simulink model "final_quadruped_080722_support_polygon"  (R2021a)
settings: Solver=ode15s  StartTime=0.0  StopTime=10  FixedStep=1e-3  RelTol=1e-5  EnableMultiTasking=on
values from neighbouring files (symbols this model uses):
  foot_x = 8    [bipedparameters.m]    (also in fcn.m; finalrobotParameters.m; finalrobotParameters_110522.m; finalrobotParameters_140522.m)
  foot_y = 6    [bipedparameters.m]    (also in fcn.m; finalrobotParameters.m; finalrobotParameters_110522.m; finalrobotParameters_140522.m)
  foot_z = 1    [bipedparameters.m]    (also in fcn.m; finalrobotParameters.m; finalrobotParameters_110522.m; finalrobotParameters_140522.m)
  height_plane = 0.025    [bipedparameters.m]    (also in finalrobotParameters.m; finalrobotParameters_110522.m; finalrobotParameters_140522.m; finalrobotParameters_240522.m)
  kd_ankle = 1000    [bipedparameters.m]    (also in finalrobotParameters_240522.m)
  kd_hip = 1000    [bipedparameters.m]    (also in finalrobotParameters_240522.m)
  kd_knee = 1000    [bipedparameters.m]    (also in finalrobotParameters_240522.m)
  ki_ankle = 1000    [bipedparameters.m]    (also in finalrobotParameters_240522.m)
  ki_hip = 1000    [bipedparameters.m]    (also in finalrobotParameters_240522.m)
  ki_knee = 2000    [bipedparameters.m]    (also in finalrobotParameters_240522.m)
  kp_ankle = 1000    [bipedparameters.m]    (also in finalrobotParameters_240522.m)
  kp_hip = 1000    [bipedparameters.m]    (also in finalrobotParameters_240522.m)
  kp_knee = 2000    [bipedparameters.m]    (also in finalrobotParameters_240522.m)
  lower_leg_length = 10    [bipedparameters.m]    (also in fcn.m; finalrobotParameters.m; finalrobotParameters_110522.m; finalrobotParameters_140522.m)
  plane_x = 25    [bipedparameters.m]    (also in finalrobotParameters.m; finalrobotParameters_110522.m; finalrobotParameters_140522.m; finalrobotParameters_240522.m)
  plane_y = 3    [bipedparameters.m]    (also in finalrobotParameters.m; finalrobotParameters_110522.m; finalrobotParameters_140522.m; finalrobotParameters_240522.m)
  torso_offset_x = -0.5    [bipedparameters.m]    (also in finalrobotParameters.m = 10; finalrobotParameters_110522.m = 10; finalrobotParameters_140522.m = 10; finalrobotParameters_240522.m = 10)
  torso_offset_z = -2    [bipedparameters.m]    (also in finalrobotParameters.m; finalrobotParameters_110522.m; finalrobotParameters_140522.m; finalrobotParameters_240522.m)
  torso_x = 5    [bipedparameters.m]    (also in fcn.m = 25; finalrobotParameters.m = 25; finalrobotParameters_110522.m = 25; finalrobotParameters_140522.m = 25)
  torso_y = 10    [bipedparameters.m]    (also in fcn.m = 16; finalrobotParameters.m = 16; finalrobotParameters_110522.m = 16; finalrobotParameters_140522.m = 16)
  torso_z = 8    [bipedparameters.m]    (also in fcn.m = 10; finalrobotParameters.m = 10; finalrobotParameters_110522.m = 10; finalrobotParameters_140522.m = 10)
  upper_leg_length = 10    [bipedparameters.m]    (also in fcn.m; finalrobotParameters.m; finalrobotParameters_110522.m; finalrobotParameters_140522.m)
undefined symbols (not defined in the file or in its folder): sigbuilder_block, X, Y, Z
libraries: nesl_utility x288, sm_lib x71, pid_lib x20, Contact_Forces_Lib x16, fl_lib x3
(part 9 of 9)

== matlab function final_quadruped_080722_support_polygon/Model/Left Leg Back/Subsystem/MATLAB Function4 ==
  data: ed1g input; ed2g input; ed_dg1 output; ed_dg2 output; ed3g input; ed_dg3 output; ed4g input; ad3g input; ad4g input; ed5g input; vlinks input; w_torso input; ed_dg4 output; td123 input; v_torso input; ed_dg5 output; td4 input; td5 input; rho_dotLB output
function [ed_dg1,ed_dg2,ed_dg3,ed_dg4,ed_dg5,rho_dotLB] = fcn(ed1g,ed2g,ed3g,ed4g,ad3g,ad4g, ed5g, vlinks, w_torso, td123, v_torso, td4, td5)
w0=w_torso;
w1=w0*td123(1);
w2=w1*td123(2);
w3=w2+ed3g*td123(3);
w4=w3+ed4g*td4;
w5=w4+ed5g*td5;

%e dot = omega X e
ed_dg1=cross(w1,ed1g);
ed_dg2=cross(w2,ed2g);
ed_dg3=cross(w3,ed3g);
ed_dg4=cross(w4,ed4g);
ed_dg5=cross(w5,ed5g);


vcf=zeros(3,5);
vof=zeros(3,5);
rho_dotLB=zeros(3,5,5);
vcf(:,1)=0;
vcf(:,2)=0;
vcf(:,3)=vlinks(10);
vcf(:,4)=vlinks(11);
vcf(:,5)=vlinks(12);
vof(:,1)=0;
vof(:,2)=0;
vof(:,3)=v_torso;
vof(:,4)=vof(:,3)+cross(w3,ad3g);
vof(:,5)=vof(:,4)+cross(w4,ad4g);
for i=1:5
    for j=1:5
        if j<i
rho_dotLB(:,j,i)=zeros(3,1);
        else
rho_dotLB(:,j,i)=vcf(:,j)-vof(:,i);
        end
    end
end

end

== matlab function final_quadruped_080722_support_polygon/Subsystem/MATLAB Function1 ==
  data: plinks input; alinks input; I3 input; I4 input; I5 input; blinks input; zmpx output; zmpy output
function [zmpx,zmpy] =fcn(plinks,alinks,I3, I4, I5, blinks)
%%
lower_leg_length = 10;
upper_leg_length = 10;
density = 1000;
foot_density=2000;
leg_radius = 0.75;
foot_x = 8;
foot_y = 6;
foot_z = 1;
torso_y = 16;
torso_x = 25;
torso_z = 10;
m_ul=density*leg_radius*leg_radius*upper_leg_length*3.141592653589*0.01*0.01*0.01;
m_ll=density*leg_radius*leg_radius*lower_leg_length*3.141592653589*0.01*0.01*0.01;
m_foot=foot_density*foot_x*foot_y*foot_z*0.000001;
m_torso=density*torso_x*torso_y*torso_z*0.000001;
M=m_torso+4*(m_ul+m_ll+m_foot);
Itorso=[0.0118667 0 0;0 0.0241667 0;0 0 0.0293667];
g=9.81;
pz=0;
%%
m=[m_ul m_ll m_foot m_ul m_ll m_foot m_ul m_ll m_foot m_ul m_ll m_foot m_torso];
Iy=[I3(2,2) I4(2,2) I5(2,2) I3(2,2) I4(2,2) I5(2,2) I3(2,2) I4(2,2) I5(2,2) I3(2,2) I4(2,2) I5(2,2) Itorso(2,2)];
Ix=[I3(1,1) I4(1,1) I5(1,1) I3(1,1) I4(1,1) I5(1,1) I3(1,1) I4(1,1) I5(1,1) I3(1,1) I4(1,1) I5(1,1) Itorso(1,1)];
zmpxn=ones(1,13);%zmpx numerator
zmpxd=ones(1,13);
zmpyn=ones(1,13);
zmpyd=ones(1,13);

%Zero moment point
sxn=0;
for i=1:13
    zmpxn(i)=m(i)*((alinks(3,i)-g)*plinks(1,i)-(plinks(3,i)-pz)*alinks(1,i))-Iy(i)*blinks(2,i);
    sxn=sxn+zmpxn(i);
end

sxd=0;
for i=1:13
    zmpxd(i)=m(i)*(alinks(3,i)-g);
    sxd=sxd+zmpxd(i);
end
zmpx=sxn/sxd;


syn=0;
for i=1:13
    zmpyn(i)=m(i)*((alinks(3,i)-g)*plinks(2,i)-(plinks(3,i)-pz)*alinks(2,i))-Ix(i)*blinks(1,i);
    syn=syn+zmpyn(i);
end

syd=0;
for i=1:13
    zmpyd(i)=m(i)*(alinks(3,i)+g);
    syd=syd+zmpyd(i);
end
zmpy=syn/syd;


end

== matlab function final_quadruped_080722_support_polygon/Subsystem/MATLAB Function2 ==
  data: bulRF input; Mbcm output; bllRF input; bfRF input; bulLF input; bllLF input; bfLF input; bulRB input; bllRB input; bfRB input; bulLB input; bllLB input; bfLB input; b_torso input; blinks output; bcm output
function [Mbcm,blinks,bcm] = fcn(bulRF,bllRF,bfRF,bulLF,bllLF,bfLF,bulRB,bllRB,bfRB,bulLB,bllLB,bfLB,b_torso)
%%
lower_leg_length = 10;
upper_leg_length = 10;
density = 1000;
foot_density=2000;
leg_radius = 0.75;
foot_x = 8;
foot_y = 6;
foot_z = 1;
torso_y = 16;
torso_x = 25;
torso_z = 10;
m_ul=density*leg_radius*leg_radius*upper_leg_length*3.141592653589*0.01*0.01*0.01;
m_ll=density*leg_radius*leg_radius*lower_leg_length*3.141592653589*0.01*0.01*0.01;
m_foot=foot_density*foot_x*foot_y*foot_z*0.000001;
m_torso=density*torso_x*torso_y*torso_z*0.000001;
M=m_torso+4*(m_ul+m_ll+m_foot);
%%
Mbcm=m_torso*b_torso+(m_ul*bulRF+m_ll*bllRF+m_foot*bfRF)+(m_ul*bulLF+m_ll*bllLF+m_foot*bfLF)+(m_ul*bulRB+m_ll*bllRB+m_foot*bfRB)+(m_ul*bulLB+m_ll*bllLB+m_foot*bfLB);
blinks=[bulRF bllRF bfRF bulLF bllLF bfLF bulRB bllRB bfRB bulLB bllLB bfLB b_torso];
bcm=Mbcm/M;
end

== matlab function final_quadruped_080722_support_polygon/Model/Right Leg Front /Contact Forces /MATLAB Function1 ==
  data: n1 input; pNRF output; n2 input; n3 input; n4 input; Qd5g input; pfRF input; p1 output; p2 output; p3 output; p4 output
function [pNRF,p1,p2,p3,p4] = fcn(n1,n2,n3,n4,Qd5g,pfRF)
foot_x = 8/2;%half of foot_x
foot_y = 6/2;
foot_dim=[foot_x; foot_y; 0];
foot_dimg=Qd5g*foot_dim;
p1=[pfRF(1)+foot_dimg(1);pfRF(2)-foot_dimg(2)];
p2=[pfRF(1)-foot_dimg(1);pfRF(2)-foot_dimg(2)];
p3=[pfRF(1)+foot_dimg(1);pfRF(2)+foot_dimg(2)];
p4=[pfRF(1)-foot_dimg(1);pfRF(2)+foot_dimg(2)];
pNRF=(p1*n1+p2*n2+p3*n3+p4*n4)/(n1+n2+n3+n4);
end

== matlab function final_quadruped_080722_support_polygon/Model/Left Leg Front /Contact Forces /MATLAB Function1 ==
  data: n1 input; pNLF output; n2 input; n3 input; n4 input; Qd5g input; pfLF input; p1 output; p2 output; p3 output; p4 output
function [pNLF,p1,p2,p3,p4] = fcn(n1,n2,n3,n4,Qd5g,pfLF)
foot_x = 8/2;%half of foot_x
foot_y = 6/2;
foot_dim=[foot_x; foot_y; 0];
foot_dimg=Qd5g*foot_dim;
p1=[pfLF(1)+foot_dimg(1);pfLF(2)-foot_dimg(2)];
p2=[pfLF(1)-foot_dimg(1);pfLF(2)-foot_dimg(2)];
p3=[pfLF(1)+foot_dimg(1);pfLF(2)+foot_dimg(2)];
p4=[pfLF(1)-foot_dimg(1);pfLF(2)+foot_dimg(2)];
pNLF=(p1*n1+p2*n2+p3*n3+p4*n4)/(n1+n2+n3+n4);
end

== matlab function final_quadruped_080722_support_polygon/Model/Right Leg Front /Subsystem/MATLAB Function ==
  data: ea1g output; ea2g output; ea3g output; ea4g output; ea5g output; aa1g output; aa2g output; qhaz input; qhax input; qhay input; qaa input; Qquat input; qka input; aa3g output; aa4g output; cma1g output; cma2g output; cma3g output; cma4g output; cma5g output; Qd5g output; I1 output; I2 output; I3 output; I4 output; I5 output
function [ea1g,ea2g,ea3g,ea4g,ea5g,aa1g,aa2g,aa3g,aa4g,cma1g,cma2g,cma3g,cma4g,cma5g,Qd5g,I1,I2,I3,I4,I5] = fcn(qhaz,qhax,qhay,qaa,Qquat,qka)
%%
lower_leg_length = 10;
upper_leg_length = 10;
foot_offset=[-1; 0; 0];
I1l=zeros(3,3);
I2l=zeros(3,3);
I3l=[1.49747e-05 0 0;
    0 1.49747e-05 0;
    0 0 4.9701e-07];
I4l=[1.49747e-05 0 0;
    0 1.49747e-05 0;
    0 0 4.9701e-07];
I5l=[0 0 2.96e-05;
    0 5.2e-05 0;
    0 0 8e-05];

%%
Qd0g=quat2rotm([Qquat(1) Qquat(2) Qquat(3) Qquat(4)]);

%x,y,z are with respect to joint's frame
%z of joint is y of robot
Qd30z=[cos(qhaz) -sin(qhaz) 0;
      sin(qhaz) cos(qhaz) 0;
      0 0 1];
Qd30y=[cos(qhay) 0 sin(qhay);
      0 1 0 ;
      -sin(qhay) 0 cos(qhay)];
Qd30x=[1 0 0;
      0 cos(qhax) -sin(qhax) ;
      0 sin(qhax) cos(qhax)];
  
Qd30=Qd30x*Qd30y*Qd30z;
Qd3g=Qd30*Qd0g;
  
Qd43=[cos(qka) 0 sin(qka);
      0 1 0 ;
      -sin(qka) 0 cos(qka)];
  
Qd54=[1 0 0;
      0 cos(qaa) -sin(qaa);
      0 sin(qaa) cos(qaa)];
  
Qd40 = Qd43* Qd30;
Qd50=Qd54*Qd40;
Qd4g=Qd40*Qd0g;
Qd5g=Qd50*Qd0g;

%axis in local frames
ed1l=[1;0;0];
ed2l=[0;1;0];
ed3l=[0;
      0;
      1];
  
ed4l=[0;
      1;
      0];
ed5l=[0;
     1;
     0];
  
%link vector in local frame
ad3l=[0;
      0;
      -upper_leg_length];
   
ad4l=[0;
      0;
      -lower_leg_length];
         
%axis in global frames
ea1g=Qd30x*Qd0g*ed1l;
ea2g=Qd30x*Qd30y*Qd0g*ed2l;
ea3g =Qd30x*Qd30y*Qd30z*Qd0g*ed3l;
ea4g = Qd4g*ed4l;
ea5g = Qd5g*ed5l;

%link vector in global frame
aa1g=0;
aa2g=0;
aa3g = Qd3g*ad3l;
aa4g = Qd4g*ad4l;

%COM distances in base frame
cma1g=0;
cma2g=0;
cma3g=aa3g/2;
cma4g=aa4g/2;
cma5g=Qd5g*foot_offset;

%I in global frame
I1=Qd30x*Qd0g*I1l*transpose(Qd30x*Qd0g);
I2=Qd30x*Qd30y*Qd0g*I2l*transpose(Qd30x*Qd30y*Qd0g);
I3=Qd30x*Qd30y*Qd30z*Qd0g*I3l*transpose(Qd30x*Qd30y*Qd30z*Qd0g);
I4=Qd4g*I4l*transpose(Qd4g);
I5=Qd5g*I5l*transpose(Qd5g);


end

== matlab function final_quadruped_080722_support_polygon/Model/Right Leg Back/Contact Forces /MATLAB Function1 ==
  data: n1 input; pNRB output; n2 input; n3 input; n4 input; Qd5g input; pfRB input; p1 output; p2 output; p3 output; p4 output
function [pNRB,p1,p2,p3,p4] = fcn(n1,n2,n3,n4,Qd5g,pfRB)
foot_x = 8/2;%half of foot_x
foot_y = 6/2;
foot_dim=[foot_x; foot_y; 0];
foot_dimg=Qd5g*foot_dim;
p1=[pfRB(1)+foot_dimg(1);pfRB(2)-foot_dimg(2)];
p2=[pfRB(1)-foot_dimg(1);pfRB(2)-foot_dimg(2)];
p3=[pfRB(1)+foot_dimg(1);pfRB(2)+foot_dimg(2)];
p4=[pfRB(1)-foot_dimg(1);pfRB(2)+foot_dimg(2)];
pNRB=(p1*n1+p2*n2+p3*n3+p4*n4)/(n1+n2+n3+n4);
end

== matlab function final_quadruped_080722_support_polygon/Model/Left Leg Back/Contact Forces /MATLAB Function1 ==
  data: n1 input; pNLB output; n2 input; n3 input; n4 input; Qd5g input; pfLB input; p1 output; p2 output; p3 output; p4 output
function [pNLB,p1,p2,p3,p4] = fcn(n1,n2,n3,n4,Qd5g,pfLB)
foot_x = 8/2;%half of foot_x
foot_y = 6/2;
foot_dim=[foot_x; foot_y; 0];
foot_dimg=Qd5g*foot_dim;
p1=[pfLB(1)+foot_dimg(1);pfLB(2)-foot_dimg(2)];
p2=[pfLB(1)-foot_dimg(1);pfLB(2)-foot_dimg(2)];
p3=[pfLB(1)+foot_dimg(1);pfLB(2)+foot_dimg(2)];
p4=[pfLB(1)-foot_dimg(1);pfLB(2)+foot_dimg(2)];
pNLB=(p1*n1+p2*n2+p3*n3+p4*n4)/(n1+n2+n3+n4);
end

== matlab function final_quadruped_080722_support_polygon/Model/MATLAB Function5 ==
  data: pNRF input; zmp output; pNLF input; pNRB input; pNLB input; NRF input; NLF input; NRB input; NLB input; p1RF input; p2RF input; p3RF input; p4RF input; n1RF input; n2RF input; n3RF input; n4RF input; p1LF input; p2LF input; p3LF input; p4LF input; n1LF input; n2LF input; n3LF input; n4LF input; p1RB input; p2RB input; p3RB input; p4RB input; n1RB input; n2RB input; n3RB input; n4RB input; p1LB input; p2LB input; p3LB input; p4LB input; n1LB input; n2LB input; n3LB input; n4LB input; pplot output
function [zmp,pplot]  = fcn(pNRF,pNLF,pNRB,pNLB,NRF,NLF,NRB,NLB,p1RF,p2RF,p3RF,p4RF,n1RF,n2RF,n3RF,n4RF,p1LF,p2LF,p3LF,p4LF,n1LF,n2LF,n3LF,n4LF,p1RB,p2RB,p3RB,p4RB,n1RB,n2RB,n3RB,n4RB,p1LB,p2LB,p3LB,p4LB,n1LB,n2LB,n3LB,n4LB)
zmp_can=(pNRF*NRF+pNLF*NLF+pNRB*NRB+pNLB*NLB)/(NRF+NLF+NRB+NLB);
zmp=(p1RF*n1RF+p2RF*n2RF+p3RF*n3RF+p4RF*n4RF+p1LF*n1LF+p2LF*n2LF+p3LF*n3LF+p4LF*n4LF+p1RB*n1RB+p2RB*n2RB+p3RB*n3RB+p4RB*n4RB+p1LB*n1LB+p2LB*n2LB+p3LB*n3LB+p4LB*n4LB)/(n1RF+n2RF+n3RF+n4RF+n1LF+n2LF+n3LF+n4LF+n1RB+n2RB+n3RB+n4RB+n1LB+n2LB+n3LB+n4LB);
N=[n1RF n2RF n3RF n4RF n1LF n2LF n3LF n4LF n1RB n2RB n3RB n4RB n1LB n2LB n3LB n4LB];
pN=[p1RF p2RF p3RF p4RF p1LF p2LF p3LF p4LF p1RB p2RB p3RB p4RB p1LB p2LB p3LB p4LB];
Nplot=[];
plotnum=[];
Nzero=[];
zero=[];
for i=1:16
    if abs(N(i))>1e-5
        Nplot=[Nplot, N(i)];
        plotnum=[plotnum, i];
        
    else
        Nzero=[Nzero, N(i)];
        zero=[zero,i];
    end
end
pplot=zeros(2,16);
for i=1:length(plotnum)
   % pplot=[pplot,pN(:,plotnum(i))];
   pplot(:,i)=pN(:,plotnum(i));
end
end

== matlab function final_quadruped_080722_support_polygon/Model/Left Leg Front /Contact Forces /MATLAB Function ==
  data: n1 input; NRF output; n2 input; n4 input; n3 input; f1 input; f2 input; f3 input; f4 input; FRF output; Qd3g input
function [NRF,FRF] = fcn(n1,n2,n4,n3,f1,f2,f3,f4, Qd3g)
% mu_s = 0.8;
% alpha=atan(mu_s);
% NRF=n1+n2+n3+n4;
% FRFca=f1*cos(alpha)+f2*cos(alpha)+f3*cos(alpha)+f4*cos(alpha);
% FRFsa=f1*sin(alpha)+f2*sin(alpha)+f3*sin(alpha)+f4*sin(alpha);
Qds3=[1 0 0;
      0 cos(90) -sin(90);
      0 sin(90) cos(90)];
NRF=n1+n2+n3+n4;
FRFl=f1+f2+f3+f4;
FRF=Qds3*Qd3g*FRFl;
end

== matlab function final_quadruped_080722_support_polygon/Model/Right Leg Back/Contact Forces /MATLAB Function ==
  data: n1 input; NRF output; n2 input; n4 input; n3 input; f1 input; f2 input; f3 input; f4 input; FRF output; Qd3g input
function [NRF,FRF] = fcn(n1,n2,n4,n3,f1,f2,f3,f4, Qd3g)
% mu_s = 0.8;
% alpha=atan(mu_s);
% NRF=n1+n2+n3+n4;
% FRFca=f1*cos(alpha)+f2*cos(alpha)+f3*cos(alpha)+f4*cos(alpha);
% FRFsa=f1*sin(alpha)+f2*sin(alpha)+f3*sin(alpha)+f4*sin(alpha);
Qds3=[1 0 0;
      0 cos(90) -sin(90);
      0 sin(90) cos(90)];
NRF=n1+n2+n3+n4;
FRFl=f1+f2+f3+f4;
FRF=Qds3*Qd3g*FRFl;
end

== matlab function final_quadruped_080722_support_polygon/Model/Left Leg Back/Contact Forces /MATLAB Function ==
  data: n1 input; NRF output; n2 input; n4 input; n3 input; f1 input; f2 input; f3 input; f4 input; FRF output; Qd3g input
function [NRF,FRF] = fcn(n1,n2,n4,n3,f1,f2,f3,f4, Qd3g)
% mu_s = 0.8;
% alpha=atan(mu_s);
% NRF=n1+n2+n3+n4;
% FRFca=f1*cos(alpha)+f2*cos(alpha)+f3*cos(alpha)+f4*cos(alpha);
% FRFsa=f1*sin(alpha)+f2*sin(alpha)+f3*sin(alpha)+f4*sin(alpha);
Qds3=[1 0 0;
      0 cos(90) -sin(90);
      0 sin(90) cos(90)];
NRF=n1+n2+n3+n4;
FRFl=f1+f2+f3+f4;
FRF=Qds3*Qd3g*FRFl;
end

== matlab function final_quadruped_080722_support_polygon/Model/MATLAB Function4 ==
  data: hLF input; hRB input; hLB input; h_dotLF input; N input; hRF input; h_dotRF input; tddRF output; v_torso input; tddLF output; tddRB output; tddLB output; h output; h_dot output; h_dotRB input; t2d input; h_dotLB input; theta_d_des output; M output; t input; alpRF input; alpLF input; alpRB input; alpLB input; alp output; x output
function [tddRF,tddLF,tddRB,tddLB,h,h_dot,theta_d_des,M,alp,x] = fcn(hLF, hRB,hLB, h_dotLF, N, hRF,h_dotRF, v_torso, h_dotRB,t2d, h_dotLB,t,alpRF,alpLF,alpRB,alpLB)
%%
lower_leg_length = 10;
upper_leg_length = 10;
density = 1000;
foot_density=2000;
leg_radius = 0.75;
foot_x = 8;
foot_y = 6;
foot_z = 1;
torso_y = 16;
torso_x = 25;
torso_z = 10;
m_ul=density*leg_radius*leg_radius*upper_leg_length*3.141592653589*0.01*0.01*0.01;
m_ll=density*leg_radius*leg_radius*lower_leg_length*3.141592653589*0.01*0.01*0.01;
m_foot=foot_density*foot_x*foot_y*foot_z*0.000001;
m_torso=density*torso_x*torso_y*torso_z*0.000001;
M=m_torso+(4*(m_ul+m_ll+m_foot));
mu_s = 0.8;
%%
h=[hRF hLF hRB hLB];
h_dot=[h_dotRF h_dotLF h_dotRB h_dotLB];
alp=[alpRF alpLF alpRB alpLB]; 

if t<0.05
    tddfun= @(x)norm(pinv(h)*(M*[x;0;0]-M*v_torso))^2+norm(alp*pinv(h)*(M*[x;0;0]-M*v_torso))^2;
    C=[1 0 0];
    A = C*h_dot*pinv(h)*pinv(C)*M;
    b = mu_s*N-N+C*h_dot*pinv(h)*pinv(C)*C*v_torso*M-C*h*t2d;
    Aeq = [];
    beq = [];
    lb = 0;
    ub =1;
    x0 = 0.001;
    options=optimoptions('fmincon', 'Algorithm', 'sqp');
    x= fmincon(tddfun,x0,A,b,[],[],lb,ub,[],options);
else
     x=0.001;
end        
% if t<0.05
%      theta_d_des=-pinv(h)*M*v_torso;
% else
%  theta_d_des=pinv(h)*(M*[x;0;0]-M*v_torso);
% end
%theta_d_des=pinv(h)*(-M*v_torso);
theta_d_des=pinv(h)*(M*[x;0;0]-M*v_torso);

tddRF_hipx=theta_d_des(1);
tddRF_hipy=theta_d_des(2);
tddRF_hipz=theta_d_des(3);
tddRF_knee=theta_d_des(4);
tddRF_ankle=theta_d_des(5);
tddLF_hipx=theta_d_des(6);
tddLF_hipy=theta_d_des(7);
tddLF_hipz=theta_d_des(8);
tddLF_knee=theta_d_des(9);
tddLF_ankle=theta_d_des(10);
tddRB_hipx=theta_d_des(11);
tddRB_hipy=theta_d_des(12);
tddRB_hipz=theta_d_des(13);
tddRB_knee=theta_d_des(14);
tddRB_ankle=theta_d_des(15);
tddLB_hipx=theta_d_des(16);
tddLB_hipy=theta_d_des(17);
tddLB_hipz=theta_d_des(18);
tddLB_knee=theta_d_des(19);
tddLB_ankle=theta_d_des(20);

tddRF=[tddRF_hipx tddRF_hipy tddRF_hipz tddRF_knee tddRF_ankle];
tddLF=[tddLF_hipx tddLF_hipy tddLF_hipz tddLF_knee tddLF_ankle];
tddRB=[tddRB_hipx tddRB_hipy tddRB_hipz tddRB_knee tddRB_ankle];
tddLB=[tddLB_hipx tddLB_hipy tddLB_hipz tddLB_knee tddLB_ankle];
end

== matlab function final_quadruped_080722_support_polygon/Model/Right Leg Front /Subsystem/MATLAB Function1 ==
  data: ea10g input; ea20g input; ea30g input; ea40g input; aa10g input; aa20g input; aa30g input; cma4 input; cma3 input; cma5 input; ea50g input; aa40g input; hRF output; rhoRF output; cma1 input; cma2 input; I1 input; I2 input; I3 input; I4 input; I5 input; CMg input; alpRF output
function [hRF,rhoRF,alpRF] = fcn(ea10g,ea20g,ea30g, ea40g,aa10g,aa20g, aa30g, cma4, cma3, cma5, ea50g, aa40g,cma1,cma2,I1,I2,I3,I4,I5, CMg)
%%
lower_leg_length = 10;
upper_leg_length = 10;
density = 1000;
foot_density=2000;
leg_radius = 0.75;
foot_x = 8;
foot_y = 6;
foot_z = 1;
m_ul=density*leg_radius*leg_radius*upper_leg_length*3.141592653589*0.01*0.01*0.01;
m_ll=density*leg_radius*leg_radius*lower_leg_length*3.141592653589*0.01*0.01*0.01;
m_foot=foot_density*foot_x*foot_y*foot_z*0.000001;
m1=0;
m2=0;
%cgtolink=[torso_offset_x -torso_y/2 torso_offset_z];
%%
scf=zeros(3,5);
sof=zeros(3,5);
rhoRF=zeros(3,5,5);
scf(:,1)=[0;0;0];
scf(:,2)=[0;0;0];
scf(:,3)=cma3;
scf(:,4)=aa30g+cma4;
scf(:,5)=aa30g+aa40g+cma5;
sof(:,1)=[0;0;0];
sof(:,2)=[0;0;0];
sof(:,3)=[0;0;0];
sof(:,4)=aa30g;
sof(:,5)=aa30g+aa40g;
for i=1:5
    for j=1:5
        if j<i
rhoRF(:,j,i)=zeros(3,1);
        else
rhoRF(:,j,i)=scf(:,j)-sof(:,i);
        end
    end
end
c5=cma5-CMg;
c4=cma4-CMg;
c3=cma3-CMg;
c2=cma2-CMg;
c1=cma1-CMg;

h1=m1*(cross(ea10g,rhoRF(:,1,1)))+m2*(cross(ea10g,rhoRF(:,2,1)))+m_ul*(cross(ea10g,rhoRF(:,3,1)))+m_ll*(cross(ea10g,rhoRF(:,4,1)))+m_foot*(cross(ea10g,rhoRF(:,5,1)));
h2=m2*(cross(ea20g,rhoRF(:,2,2)))+m_ul*(cross(ea20g,rhoRF(:,3,2)))+m_ll*(cross(ea20g,rhoRF(:,4,2)))+m_foot*(cross(ea20g,rhoRF(:,5,2)));
h3=(m_ul*cross(ea30g,rhoRF(:,3,3)))+(m_ll*cross(ea30g,rhoRF(:,4,3)))+(m_foot*cross(ea30g,rhoRF(:,5,3)));
h4=(m_ll*cross(ea40g,rhoRF(:,4,4)))+(m_foot*cross(ea40g,rhoRF(:,5,4)));
h5=m_foot*(cross(ea50g,rhoRF(:,5,5)));

hRF =[h1 h2 h3 h4 h5];

alp1=skewsymmetric(c1)*m1*cross(ea10g,rhoRF(:,1,1))+skewsymmetric(c2)*m2*cross(ea10g,rhoRF(:,2,1))+skewsymmetric(c3)*m_ul*cross(ea10g,rhoRF(:,3,1))+skewsymmetric(c4)*m_ll*cross(ea10g,rhoRF(:,4,1))+skewsymmetric(c5)*m_foot*cross(ea10g,rhoRF(:,5,1))+(I1+I2+I3+I4+I5)*ea10g;
alp2=skewsymmetric(c2)*m2*(cross(ea20g,rhoRF(:,2,2)))+skewsymmetric(c3)*m_ul*(cross(ea20g,rhoRF(:,3,2)))+skewsymmetric(c4)*m_ll*(cross(ea20g,rhoRF(:,4,2)))+skewsymmetric(c5)*m_foot*(cross(ea20g,rhoRF(:,5,2)));+(I2+I3+I4+I5)*ea20g;
alp3=skewsymmetric(c3)*m_ul*cross(ea30g,rhoRF(:,3,3))+skewsymmetric(c4)*m_ll*cross(ea30g,rhoRF(:,4,3))+skewsymmetric(c5)*m_foot*cross(ea30g,rhoRF(:,5,3))+(I3+I4+I5)*ea30g;
alp4=skewsymmetric(c4)*m_ll*cross(ea40g,rhoRF(:,4,4))+skewsymmetric(c5)*m_foot*cross(ea40g,rhoRF(:,5,4))+(I4+I5)*ea40g;
alp5=skewsymmetric(c5)*m_foot*cross(ea50g,rhoRF(:,5,5))+I5*ea50g;

alpRF=[alp1 alp2 alp3 alp4 alp5];

end

== matlab function final_quadruped_080722_support_polygon/Model/Left Leg Front /Hip/MATLAB Function ==
  data: qx input; hip output; qy input; qz input
function hip = fcn(qx,qy,qz)
hip=[qx;qy;qz];
end

== matlab function final_quadruped_080722_support_polygon/Model/Right Leg Back/Hip/MATLAB Function ==
  data: qx input; hip output; qy input; qz input
function hip = fcn(qx,qy,qz)
hip=[qx;qy;qz];
end

== matlab function final_quadruped_080722_support_polygon/Model/Left Leg Back/Hip/MATLAB Function ==
  data: qx input; hip output; qy input; qz input
function hip = fcn(qx,qy,qz)
hip=[qx;qy;qz];
end

== matlab function final_quadruped_080722_support_polygon/MATLAB Function ==
  data: vx input; v_torso output; vy input; vz input
function v_torso = fcn(vx, vy, vz)
v_torso=[vx; vy; vz];
end

== matlab function final_quadruped_080722_support_polygon/Model/Right Leg Front /MATLAB Function2 ==
  data: tddRF input; tddRF_hip output; tddRF_knee output; tddRF_ankle output
function [tddRF_hip, tddRF_knee, tddRF_ankle] = fcn(tddRF)
tddRF_hip=[tddRF(1);tddRF(2);tddRF(3)];
tddRF_knee=tddRF(4);
tddRF_ankle=tddRF(5);
end

== matlab function final_quadruped_080722_support_polygon/Model/Left Leg Front /Hip/MATLAB Function1 ==
  data: wx input; hip output; wy input; wz input
function hip = fcn(wx,wy,wz)
hip=[wx;wy;wz];
end

== matlab function final_quadruped_080722_support_polygon/Model/Right Leg Back/Hip/MATLAB Function1 ==
  data: wx input; hip output; wy input; wz input
function hip = fcn(wx,wy,wz)
hip=[wx;wy;wz];
end

== matlab function final_quadruped_080722_support_polygon/Model/Left Leg Back/Hip/MATLAB Function1 ==
  data: wx input; hip output; wy input; wz input
function hip = fcn(wx,wy,wz)
hip=[wx;wy;wz];
end

== matlab function final_quadruped_080722_support_polygon/Subsystem/LF/MATLAB Function4 ==
  data: b output; bx input; by input; bz input; px input; py input; pz input; p output; vx input; vy input; v output; vz input; ax input; ay input; az input; a output
function [b,p,v,a] = fcn(bx,by,bz,px,py,pz,vx,vy,vz,ax,ay,az)
b=[bx;by;bz];
p=[px;py;pz];
v=[vx;vy;vz];
a=[ax;ay;az];
end

== matlab function final_quadruped_080722_support_polygon/Subsystem/RB/MATLAB Function5 ==
  data: bx input; by input; bz input; b output; px input; py input; pz input; p output; vx input; vy input; v output; vz input; ax input; ay input; az input; a output
function [b,p,v,a] = fcn(bx,by,bz,px,py,pz,vx,vy,vz,ax,ay,az)
b=[bx;by;bz];
p=[px;py;pz];
v=[vx;vy;vz];
a=[ax;ay;az];
end

== matlab function final_quadruped_080722_support_polygon/Subsystem/RB/MATLAB Function6 ==
  data: bx input; by input; bz input; b output; px input; py input; pz input; p output; vx input; vy input; v output; vz input; ax input; ay input; az input; a output
function [b,p,v,a] = fcn(bx,by,bz,px,py,pz,vx,vy,vz,ax,ay,az)
b=[bx;by;bz];
p=[px;py;pz];
v=[vx;vy;vz];
a=[ax;ay;az];
end

== matlab function final_quadruped_080722_support_polygon/Subsystem/RB/MATLAB Function7 ==
  data: bx input; by input; bz input; b output; px input; py input; pz input; p output; vx input; vy input; v output; vz input; ax input; ay input; az input; a output
function [b,p,v,a] = fcn(bx,by,bz,px,py,pz,vx,vy,vz,ax,ay,az)
p=[px;py;pz];
v=[vx;vy;vz];
a=[ax;ay;az];
b=[bx;by;bz];
end

== matlab function final_quadruped_080722_support_polygon/Subsystem/LF/MATLAB Function8 ==
  data: bx input; by input; bz input; b output; px input; py input; pz input; p output; vx input; vy input; v output; vz input; ax input; ay input; az input; a output
function [b,p,v,a] = fcn(bx,by,bz,px,py,pz,vx,vy,vz,ax,ay,az)
b=[bx;by;bz];
p=[px;py;pz];
v=[vx;vy;vz];
a=[ax;ay;az];
end

== matlab function final_quadruped_080722_support_polygon/Subsystem/LB/MATLAB Function9 ==
  data: bx input; by input; bz input; b output; px input; py input; pz input; p output; vx input; vy input; v output; vz input; ax input; ay input; az input; a output
function [b,p,v,a] = fcn(bx,by,bz,px,py,pz,vx,vy,vz,ax,ay,az)
b=[bx;by;bz];
p=[px;py;pz];
v=[vx;vy;vz];
a=[ax;ay;az];
end

== matlab function final_quadruped_080722_support_polygon/Subsystem/LB/MATLAB Function10 ==
  data: bx input; by input; bz input; b output; px input; py input; pz input; p output; vx input; vy input; v output; vz input; ax input; ay input; az input; a output
function [b,p,v,a] = fcn(bx,by,bz,px,py,pz,vx,vy,vz,ax,ay,az)
b=[bx;by;bz];
p=[px;py;pz];
v=[vx;vy;vz];
a=[ax;ay;az];
end

== matlab function final_quadruped_080722_support_polygon/Subsystem/ RF/MATLAB Function1 ==
  data: b output; bx input; by input; bz input; px input; py input; pz input; p output; vx input; vy input; v output; vz input; ax input; ay input; az input; a output
function [b,p,v,a] = fcn(bx,by,bz,px,py,pz,vx,vy,vz,ax,ay,az)
b=[bx;by;bz];
p=[px;py;pz];
v=[vx;vy;vz];
a=[ax;ay;az];
end

== matlab function final_quadruped_080722_support_polygon/Subsystem/LF/MATLAB Function11 ==
  data: bx input; by input; bz input; b output; px input; py input; pz input; p output; vx input; vy input; v output; vz input; ax input; ay input; az input; a output
function [b,p,v,a] = fcn(bx,by,bz,px,py,pz,vx,vy,vz,ax,ay,az)
b=[bx;by;bz];
p=[px;py;pz];
v=[vx;vy;vz];
a=[ax;ay;az];
end

== matlab function final_quadruped_080722_support_polygon/Subsystem/LB/MATLAB Function12 ==
  data: bx input; by input; bz input; b output; px input; py input; pz input; p output; vx input; vy input; v output; vz input; ax input; ay input; az input; a output
function [b,p,v,a] = fcn(bx,by,bz,px,py,pz,vx,vy,vz,ax,ay,az)
b=[bx;by;bz];
p=[px;py;pz];
v=[vx;vy;vz];
a=[ax;ay;az];
end

== matlab function final_quadruped_080722_support_polygon/Subsystem/MATLAB Function14 ==
  data: bx input; by input; bz input; b output; px input; py input; pz input; p output; vx input; vy input; v output; vz input; ax input; ay input; az input; a output
function [b,p,v,a] = fcn(bx,by,bz,px,py,pz,vx,vy,vz,ax,ay,az)
b=[bx;by;bz];
p=[px;py;pz];
v=[vx;vy;vz];
a=[ax;ay;az];
end

== matlab function final_quadruped_080722_support_polygon/Model/Right Leg Front /MATLAB Function ==
  data: ankle input; knee input; tdRF output; hip input
function tdRF= fcn(ankle, knee, hip)
tdRF=[hip;knee;ankle];
end

== matlab function final_quadruped_080722_support_polygon/Model/Left Leg Front /Hip/MATLAB Function2 ==
  data: tddRF input; tddRFx output; tddRFy output; tddRFz output
function [tddRFx,tddRFy,tddRFz] = fcn(tddRF)
tddRFx=tddRF(1);
tddRFy=tddRF(2);
tddRFz=tddRF(3);
end

== matlab function final_quadruped_080722_support_polygon/Model/Right Leg Back/Hip/MATLAB Function2 ==
  data: tddRF input; tddRFx output; tddRFy output; tddRFz output
function [tddRFx,tddRFy,tddRFz] = fcn(tddRF)
tddRFx=tddRF(1);
tddRFy=tddRF(2);
tddRFz=tddRF(3);
end

== matlab function final_quadruped_080722_support_polygon/Model/Left Leg Back/Hip/MATLAB Function2 ==
  data: tddRF input; tddRFx output; tddRFy output; tddRFz output
function [tddRFx,tddRFy,tddRFz] = fcn(tddRF)
tddRFx=tddRF(1);
tddRFy=tddRF(2);
tddRFz=tddRF(3);
end

== matlab function final_quadruped_080722_support_polygon/Model/MATLAB Function ==
  data: tdRF input; td output; tdLF input; tdRB input; tdLB input; t2dRF input; t2dLF input; t2dRB input; t2dLB input; t2d output
function [td,t2d] = fcn(tdRF,tdLF,tdRB,tdLB,t2dRF,t2dLF,t2dRB,t2dLB)
td=[tdRF;tdLF;tdRB;tdLB];
t2d=[t2dRF;t2dLF;t2dRB;t2dLB];
end

== matlab function final_quadruped_080722_support_polygon/Model/MATLAB Function1 ==
  data: h input; h_dot input; ht2d output; td input; t2d input; h_dottd output; htd output; theta_d_des input; theta_2d_des input; ht2ddes output; hdtddes output
function [ht2d,h_dottd,htd,ht2ddes,hdtddes] = fcn(h,h_dot, td, t2d,theta_d_des,theta_2d_des)
ht2d=h*t2d;
htd=h*td;
h_dottd=h_dot*td;
ht2ddes=h*theta_2d_des;
hdtddes=h_dot*theta_d_des;
end

== matlab function final_quadruped_080722_support_polygon/MATLAB Function1 ==
  data: Mvcm input; v_error_des output; ht2d input; h_dottd input; a_torso input; v_torso input; f input; Macm input; htd input; ht2ddes input; hdtddes input; theta_d_des input; h input; v_error_act output
function [v_error_des,v_error_act] = fcn(Mvcm,ht2d,h_dottd,a_torso, v_torso, f,Macm,htd, ht2ddes, hdtddes, theta_d_des,h)
%%
lower_leg_length = 10;
upper_leg_length = 10;
density = 1000;
foot_density=2000;
leg_radius = 0.75;
foot_x = 8;
foot_y = 6;
foot_z = 1;
torso_y = 16;
torso_x = 25;
torso_z = 10;
m_ul=density*leg_radius*leg_radius*upper_leg_length*3.141592653589*0.01*0.01*0.01;
m_ll=density*leg_radius*leg_radius*lower_leg_length*3.141592653589*0.01*0.01*0.01;
m_foot=foot_density*foot_x*foot_y*foot_z*0.000001;
m_torso=density*torso_x*torso_y*torso_z*0.000001;
M=m_torso+(4*(m_ul+m_ll+m_foot));
g=[0; 0; -9.80067];
%%
%v_error=htd+M*v_torso-Mvcm;
v_error_des=h*theta_d_des+M*v_torso-Mvcm;
v_error_act=htd+M*v_torso-Mvcm;
%v_error_eig=h*theta_d_des+M*v_torso-Mvcm;
%error2=ht2d+h_dottd+M*a_torso-M*g-f-Macm;
%error=ht2ddes+hdtddes+M*a_torso-M*g-f-Macm;
end

== matlab function final_quadruped_080722_support_polygon/Model/Right Leg Front /Subsystem/MATLAB Function2 ==
  data: ea1g input; ea2g input; h_dotRF output; ea_dg1 input; ea_dg2 input; ea_dg3 input; ea3g input; ea4g input; ea5g input; ea_dg4 input; ea_dg5 input; rho_dotRF input; rhoRF input
function h_dotRF = fcn( ea1g,ea2g,ea_dg1,ea_dg2,ea_dg3,ea3g, ea4g, ea5g, ea_dg4, ea_dg5, rho_dotRF, rhoRF)
%%
lower_leg_length = 10;
upper_leg_length = 10;
density = 1000;
foot_density=2000;
leg_radius = 0.75;
foot_x = 8;
foot_y = 6;
foot_z = 1;
m_ul=density*leg_radius*leg_radius*upper_leg_length*3.141592653589*0.01*0.01*0.01;
m_ll=density*leg_radius*leg_radius*lower_leg_length*3.141592653589*0.01*0.01*0.01;
m_foot=foot_density*foot_x*foot_y*foot_z*0.000001;
m1=0;
m2=0;
%%
h1_dot=m1*(cross(ea1g,rho_dotRF(:,1,1)))+m1*(cross(ea_dg1,rhoRF(:,1,1)))+m2*(cross(ea1g,rho_dotRF(:,2,1)))+m2*(cross(ea_dg1,rhoRF(:,2,1)))+m_ul*(cross(ea1g,rho_dotRF(:,3,1)))+m_ul*(cross(ea_dg1,rhoRF(:,3,1)))+m_ll*(cross(ea1g,rho_dotRF(:,4,1)))+m_ll*(cross(ea_dg1,rhoRF(:,4,1)))+m_foot*(cross(ea1g,rho_dotRF(:,5,1)))+m_foot*(cross(ea_dg1,rhoRF(:,5,1)));
h2_dot=m2*(cross(ea2g,rho_dotRF(:,2,2)))+m2*(cross(ea_dg2,rhoRF(:,2,2)))+m_ul*(cross(ea2g,rho_dotRF(:,3,2)))+m_ul*(cross(ea_dg2,rhoRF(:,3,2)))+m_ll*(cross(ea2g,rho_dotRF(:,4,2)))+m_ll*(cross(ea_dg2,rhoRF(:,4,2)))+m_foot*(cross(ea2g,rho_dotRF(:,5,2)))+m_foot*(cross(ea_dg2,rhoRF(:,5,2)));
h3_dot=(m_ul*cross(ea3g,rho_dotRF(:,3,3)))+(m_ul*cross(ea_dg3,rhoRF(:,3,3)))+(m_ll*cross(ea3g,rho_dotRF(:,4,3)))+(m_ll*cross(ea_dg3,rhoRF(:,4,3)))+(m_foot*cross(ea3g,rho_dotRF(:,5,3)))+(m_foot*cross(ea_dg3,rhoRF(:,5,3)));
h4_dot=(m_ll*cross(ea4g,rho_dotRF(:,4,4)))+(m_ll*cross(ea_dg4,rhoRF(:,4,4)))+(m_foot*cross(ea4g,rho_dotRF(:,5,4)))+(m_foot*cross(ea_dg4,rhoRF(:,5,4)));
h5_dot=m_foot*(cross(ea5g,rho_dotRF(:,5,5)))+m_foot*(cross(ea_dg5,rhoRF(:,5,5)));

h_dotRF =[h1_dot h2_dot h3_dot h4_dot h5_dot];



end

== matlab function final_quadruped_080722_support_polygon/Model/Left Leg Front /Hip/MATLAB Function3 ==
  data: bx input; hip output; by input; bz input
function hip = fcn(bx,by,bz)
hip=[bx;by;bz];
end

== matlab function final_quadruped_080722_support_polygon/Model/Right Leg Front /Subsystem/MATLAB Function4 ==
  data: ea1g input; ea2g input; ea_dg1 output; ea_dg2 output; ea3g input; ea_dg3 output; ea4g input; aa3g input; aa4g input; ea5g input; vlinks input; w_torso input; ea_dg4 output; td123 input; v_torso input; ea_dg5 output; td4 input; td5 input; rho_dotRF output
function [ea_dg1,ea_dg2,ea_dg3,ea_dg4,ea_dg5,rho_dotRF] = fcn(ea1g,ea2g,ea3g,ea4g,aa3g,aa4g, ea5g, vlinks, w_torso, td123, v_torso, td4, td5)
w0=w_torso;
w1=w0*td123(1);
w2=w1*td123(2);
w3=w2+ea3g*td123(3);
w4=w3+ea4g*td4;
w5=w4+ea5g*td5;

%e dot = omega X e
ea_dg1=cross(w1,ea1g);
ea_dg2=cross(w2,ea2g);
ea_dg3=cross(w3,ea3g);
ea_dg4=cross(w4,ea4g);
ea_dg5=cross(w5,ea5g);


vcf=zeros(3,5);
vof=zeros(3,5);
rho_dotRF=zeros(3,5,5);
vcf(:,1)=0;
vcf(:,2)=0;
vcf(:,3)=vlinks(1);
vcf(:,4)=vlinks(2);
vcf(:,5)=vlinks(3);
vof(:,1)=0;
vof(:,2)=0;
vof(:,3)=v_torso;
vof(:,4)=vof(:,3)+cross(w3,aa3g);
vof(:,5)=vof(:,4)+cross(w4,aa4g);
for i=1:5
    for j=1:5
        if j<i
rho_dotRF(:,j,i)=zeros(3,1);
        else
rho_dotRF(:,j,i)=vcf(:,j)-vof(:,i);
        end
    end
end

end

== matlab function final_quadruped_080722_support_polygon/Model/Left Leg Front /MATLAB Function ==
  data: ankle input; knee input; tdLF output; hip input
function tdLF= fcn(ankle, knee, hip)
tdLF=[hip;knee;ankle];
end

== matlab function final_quadruped_080722_support_polygon/Subsystem/MATLAB Function13 ==
  data: vulRF input; vllRF input; Mvcm output; vfRF input; vulLF input; vllLF input; vfLF input; vulRB input; vllRB input; vfRB input; vulLB input; vllLB input; vfLB input; v_torso input; vlinks output; vcm output
function [Mvcm,vlinks,vcm] = fcn(vulRF,vllRF,vfRF,vulLF,vllLF,vfLF,vulRB,vllRB,vfRB,vulLB,vllLB,vfLB,v_torso)
%%
lower_leg_length = 10;
upper_leg_length = 10;
density = 1000;
foot_density=2000;
leg_radius = 0.75;
foot_x = 8;
foot_y = 6;
foot_z = 1;
torso_y = 16;
torso_x = 25;
torso_z = 10;
m_ul=density*leg_radius*leg_radius*upper_leg_length*3.141592653589*0.01*0.01*0.01;
m_ll=density*leg_radius*leg_radius*lower_leg_length*3.141592653589*0.01*0.01*0.01;
m_foot=foot_density*foot_x*foot_y*foot_z*0.000001;
m_torso=density*torso_x*torso_y*torso_z*0.000001;
M=m_torso+4*(m_ul+m_ll+m_foot);
%%
Mvcm=m_torso*v_torso+(m_ul*vulRF+m_ll*vllRF+m_foot*vfRF)+(m_ul*vulLF+m_ll*vllLF+m_foot*vfLF)+(m_ul*vulRB+m_ll*vllRB+m_foot*vfRB)+(m_ul*vulLB+m_ll*vllLB+m_foot*vfLB);
vlinks=[vulRF vllRF vfRF vulLF vllLF vfLF vulRB vllRB vfRB vulLB vllLB vfLB v_torso];
vcm=Mvcm/M;
end

== matlab function final_quadruped_080722_support_polygon/Model/Right Leg Back/Hip/MATLAB Function3 ==
  data: bx input; hip output; by input; bz input
function hip = fcn(bx,by,bz)
hip=[bx;by;bz];
end

== matlab function final_quadruped_080722_support_polygon/Model/Right Leg Back/MATLAB Function ==
  data: ankle input; knee input; tdRB output; hip input
function tdRB= fcn(ankle, knee, hip)
tdRB=[hip;knee;ankle];
end

== matlab function final_quadruped_080722_support_polygon/Model/Left Leg Back/Hip/MATLAB Function3 ==
  data: bx input; hip output; by input; bz input
function hip = fcn(bx,by,bz)
hip=[bx;by;bz];
end

== matlab function final_quadruped_080722_support_polygon/Model/Left Leg Back/MATLAB Function ==
  data: ankle input; knee input; tdLB output; hip input
function tdLB= fcn(ankle, knee, hip)
tdLB=[hip;knee;ankle];
end

== matlab function final_quadruped_080722_support_polygon/Model/Left Leg Front /MATLAB Function1 ==
  data: ankle input; knee input; t2dLF output; hip input
function t2dLF= fcn(ankle, knee, hip)
t2dLF=[hip;knee;ankle];
end

== matlab function final_quadruped_080722_support_polygon/Model/Right Leg Front /MATLAB Function1 ==
  data: ankle input; knee input; t2dRF output; hip input
function t2dRF= fcn(ankle, knee, hip)
t2dRF=[hip;knee;ankle];
end

== matlab function final_quadruped_080722_support_polygon/MATLAB Function2 ==
  data: ax input; a_torso output; ay input; az input
function a_torso = fcn(ax, ay, az)
a_torso=[ax(1); ay(1); az(1)];
end

== matlab function final_quadruped_080722_support_polygon/Model/Left Leg Front /MATLAB Function2 ==
  data: tddLF input; tddLF_hip output; tddLF_knee output; tddLF_ankle output
function [tddLF_hip, tddLF_knee, tddLF_ankle] = fcn(tddLF)
tddLF_hip=[tddLF(1);tddLF(2);tddLF(3)];
tddLF_knee=tddLF(4);
tddLF_ankle=tddLF(5);
end

== matlab function final_quadruped_080722_support_polygon/Model/MATLAB Function2 ==
  data: theta_d_des input; theta_2d_des output; h_dot input; h input; a_torso input; M input; f input
function theta_2d_des = fcn(theta_d_des, h_dot, h, a_torso, M, f)
g=[0; 0; -9.80665];
theta_2d_des=pinv(h)*((-h_dot*theta_d_des)-M*a_torso+M*g+f);
end

== matlab function final_quadruped_080722_support_polygon/Model/Right Leg Front /Contact Forces /MATLAB Function ==
  data: n1 input; NRF output; n2 input; n4 input; n3 input; f1 input; f2 input; f3 input; f4 input; FRF output; Qd5g input
function [NRF,FRF] = fcn(n1,n2,n4,n3,f1,f2,f3,f4, Qd5g)
% mu_s = 0.8;
% alpha=atan(mu_s);
% NRF=n1+n2+n3+n4;
% FRFca=f1*cos(alpha)+f2*cos(alpha)+f3*cos(alpha)+f4*cos(alpha);
% FRFsa=f1*sin(alpha)+f2*sin(alpha)+f3*sin(alpha)+f4*sin(alpha);
Qds3=[1 0 0;
      0 cos(90) -sin(90);
      0 sin(90) cos(90)];
NRF=n1+n2+n3+n4;
FRFl=f1+f2+f3+f4;
FRF=Qds3*Qd5g*FRFl;
end

== matlab function final_quadruped_080722_support_polygon/Model/Right Leg Back/MATLAB Function1 ==
  data: ankle input; knee input; t2dRB output; hip input
function t2dRB= fcn(ankle, knee, hip)
t2dRB=[hip;knee;ankle];
end

== matlab function final_quadruped_080722_support_polygon/Model/Left Leg Back/MATLAB Function1 ==
  data: ankle input; knee input; t2dLB output; hip input
function t2dLB= fcn(ankle, knee, hip)
t2dLB=[hip;knee;ankle];
end

== matlab function final_quadruped_080722_support_polygon/Model/MATLAB Function3 ==
  data: NRF input; f output; FRF input; NLF input; FLF input; NRB input; FRB input; NLB input; FLB input; N output
function [f,N] = fcn(NRF,FRF,NLF,FLF,NRB,FRB, NLB,FLB)
N=NRF+NLF+NRB+NLB;
F=FRF+FLF+FRB+FLB;
f=[-F(1);-F(2); N+F(3)];
end

== matlab function final_quadruped_080722_support_polygon/Model/Right Leg Front /MATLAB Function3 ==
  data: theta_2d_des input; t2ddhip output; t2ddknee output; t2ddankle output
function [t2ddhip,t2ddknee,t2ddankle] = fcn(theta_2d_des)
t2ddhip=theta_2d_des(1);
t2ddknee=theta_2d_des(2);
t2ddankle=theta_2d_des(3);

end

== matlab function final_quadruped_080722_support_polygon/Model/Left Leg Front /MATLAB Function3 ==
  data: theta_2d_des input; t2ddhip output; t2ddknee output; t2ddankle output
function [t2ddhip,t2ddknee,t2ddankle] = fcn(theta_2d_des)
t2ddhip=theta_2d_des(8);
t2ddknee=theta_2d_des(9);
t2ddankle=theta_2d_des(10);

end

== matlab function final_quadruped_080722_support_polygon/Model/Right Leg Back/MATLAB Function2 ==
  data: tddRB input; tddRB_hip output; tddRB_knee output; tddRB_ankle output
function [tddRB_hip, tddRB_knee, tddRB_ankle] = fcn(tddRB)
tddRB_hip=[tddRB(1);tddRB(2);tddRB(3)];
tddRB_knee=tddRB(4);
tddRB_ankle=tddRB(5);
end

== matlab function final_quadruped_080722_support_polygon/Model/Left Leg Back/MATLAB Function2 ==
  data: tddLB input; tddLB_hip output; tddLB_knee output; tddLB_ankle output
function [tddLB_hip, tddLB_knee, tddLB_ankle] = fcn(tddLB)
tddLB_hip=[tddLB(1);tddLB(2);tddLB(3)];
tddLB_knee=tddLB(4);
tddLB_ankle=tddLB(5);
end

== matlab function final_quadruped_080722_support_polygon/Model/Right Leg Back/MATLAB Function3 ==
  data: theta_2d_des input; t2ddhip output; t2ddknee output; t2ddankle output
function [t2ddhip,t2ddknee,t2ddankle] = fcn(theta_2d_des)
t2ddhip=theta_2d_des(1);
t2ddknee=theta_2d_des(2);
t2ddankle=theta_2d_des(3);

end

== matlab function final_quadruped_080722_support_polygon/Model/Left Leg Back/MATLAB Function3 ==
  data: theta_2d_des input; t2ddhip output; t2ddknee output; t2ddankle output
function [t2ddhip,t2ddknee,t2ddankle] = fcn(theta_2d_des)
t2ddhip=theta_2d_des(8);
t2ddknee=theta_2d_des(9);
t2ddankle=theta_2d_des(10);

end

== matlab function final_quadruped_080722_support_polygon/Subsystem/MATLAB Function ==
  data: aulRF input; Macm output; allRF input; afRF input; aulLF input; allLF input; afLF input; aulRB input; allRB input; afRB input; aulLB input; allLB input; afLB input; a_torso input; alinks output; acm output
function [Macm,alinks,acm] = fcn(aulRF,allRF,afRF,aulLF,allLF,afLF,aulRB,allRB,afRB,aulLB,allLB,afLB,a_torso)
%%
lower_leg_length = 10;
upper_leg_length = 10;
density = 1000;
foot_density=2000;
leg_radius = 0.75;
foot_x = 8;
foot_y = 6;
foot_z = 1;
torso_y = 16;
torso_x = 25;
torso_z = 10;
m_ul=density*leg_radius*leg_radius*upper_leg_length*3.141592653589*0.01*0.01*0.01;
m_ll=density*leg_radius*leg_radius*lower_leg_length*3.141592653589*0.01*0.01*0.01;
m_foot=foot_density*foot_x*foot_y*foot_z*0.000001;
m_torso=density*torso_x*torso_y*torso_z*0.000001;
M=m_torso+4*(m_ul+m_ll+m_foot);
%%
Macm=m_torso*a_torso+(m_ul*aulRF+m_ll*allRF+m_foot*afRF)+(m_ul*aulLF+m_ll*allLF+m_foot*afLF)+(m_ul*aulRB+m_ll*allRB+m_foot*afRB)+(m_ul*aulLB+m_ll*allLB+m_foot*afLB);
alinks=[aulRF allRF afRF aulLF allLF afLF aulRB allRB afRB aulLB allLB afLB a_torso];
acm=Macm/M;
end

== matlab function final_quadruped_080722_support_polygon/Subsystem/ RF/MATLAB Function2 ==
  data: b output; bx input; by input; bz input; px input; py input; pz input; p output; vx input; vy input; v output; vz input; ax input; ay input; az input; a output
function [b,p,v,a] = fcn(bx,by,bz,px,py,pz,vx,vy,vz,ax,ay,az)
b=[bx;by;bz];
p=[px;py;pz];
v=[vx;vy;vz];
a=[ax;ay;az];
end

== matlab function final_quadruped_080722_support_polygon/Subsystem/MATLAB Function15 ==
  data: pulRF input; pllRF input; pfRF input; pulLF input; pllLF input; pfLF input; pulRB input; pllRB input; pfRB input; pulLB input; pllLB input; pfLB input; p_torso input; pcm output; plinks output
function [pcm,plinks] = fcn(pulRF,pllRF,pfRF,pulLF,pllLF,pfLF,pulRB,pllRB,pfRB,pulLB,pllLB,pfLB,p_torso)
%%
lower_leg_length = 10;
upper_leg_length = 10;
density = 1000;
foot_density=2000;
leg_radius = 0.75;
foot_x = 8;
foot_y = 6;
foot_z = 1;
torso_y = 16;
torso_x = 25;
torso_z = 10;
m_ul=density*leg_radius*leg_radius*upper_leg_length*3.141592653589*0.01*0.01*0.01;
m_ll=density*leg_radius*leg_radius*lower_leg_length*3.141592653589*0.01*0.01*0.01;
m_foot=foot_density*foot_x*foot_y*foot_z*0.000001;
m_torso=density*torso_x*torso_y*torso_z*0.000001;
M=m_torso+4*(m_ul+m_ll+m_foot);
%%
Mpcm=m_torso*p_torso+(m_ul*pulRF+m_ll*pllRF+m_foot*pfRF)+(m_ul*pulLF+m_ll*pllLF+m_foot*pfLF)+(m_ul*pulRB+m_ll*pllRB+m_foot*pfRB)+(m_ul*pulLB+m_ll*pllLB+m_foot*pfLB);
plinks=[pulRF pllRF pfRF pulLF pllLF pfLF pulRB pllRB pfRB pulLB pllLB pfLB p_torso];
pcm=Mpcm/M;
end

== matlab function final_quadruped_080722_support_polygon/Model/Right Leg Front /Hip/MATLAB Function ==
  data: qx input; hip output; qy input; qz input
function hip = fcn(qx,qy,qz)
hip=[qx;qy;qz];
end

== matlab function final_quadruped_080722_support_polygon/Model/Right Leg Front /Hip/MATLAB Function1 ==
  data: wx input; hip output; wy input; wz input
function hip = fcn(wx,wy,wz)
hip=[wx;wy;wz];
end

== matlab function final_quadruped_080722_support_polygon/Model/Right Leg Front /Hip/MATLAB Function2 ==
  data: tddRF input; tddRFx output; tddRFy output; tddRFz output
function [tddRFx,tddRFy,tddRFz] = fcn(tddRF)
tddRFx=tddRF(1);
tddRFy=tddRF(2);
tddRFz=tddRF(3);
end

== matlab function final_quadruped_080722_support_polygon/Model/Right Leg Front /Hip/MATLAB Function3 ==
  data: bx input; hip output; by input; bz input
function hip = fcn(bx,by,bz)
hip=[bx;by;bz];
end

== matlab function final_quadruped_080722_support_polygon/Model/Left Leg Front /Subsystem/MATLAB Function ==
  data: eb1g output; eb2g output; eb3g output; eb4g output; eb5g output; ab1g output; ab2g output; qhbz input; qhbx input; qhby input; qab input; Qquat input; qkb input; ab3g output; ab4g output; cmb1g output; cmb2g output; cmb3g output; cmb4g output; cmb5g output; Qd5g output; I1 output; I2 output; I3 output; I4 output; I5 output
function [eb1g,eb2g,eb3g,eb4g,eb5g,ab1g,ab2g,ab3g,ab4g,cmb1g,cmb2g,cmb3g,cmb4g,cmb5g,Qd5g,I1,I2,I3,I4,I5] = fcn(qhbz,qhbx,qhby,qab,Qquat,qkb)
%%
lower_leg_length = 10;
upper_leg_length = 10;
foot_offset=[-1; 0; 0];

I1l=zeros(3,3);
I2l=zeros(3,3);
I3l=[1.49747e-05 0 0;
    0 1.49747e-05 0;
    0 0 4.9701e-07];
I4l=[1.49747e-05 0 0;
    0 1.49747e-05 0;
    0 0 4.9701e-07];
I5l=[0 0 2.96e-05;
    0 5.2e-05 0;
    0 0 8e-05];
%%
Qd0g=quat2rotm([Qquat(1) Qquat(2) Qquat(3) Qquat(4)]);

%x,y,z are with respect to joint's frame
%z of joint is y of robot
Qd30z=[cos(qhbz) -sin(qhbz) 0;
      sin(qhbz) cos(qhbz) 0;
      0 0 1];
Qd30y=[cos(qhby) 0 sin(qhby);
      0 1 0 ;
      -sin(qhby) 0 cos(qhby)];
Qd30x=[1 0 0;
      0 cos(qhbx) -sin(qhbx) ;
      0 sin(qhbx) cos(qhbx)];
  
Qd30=Qd30x*Qd30y*Qd30z;
Qd3g=Qd30*Qd0g;
  
Qd43=[cos(qkb) 0 sin(qkb);
      0 1 0 ;
      -sin(qkb) 0 cos(qkb)];
  
Qd54=[1 0 0;
      0 cos(qab) -sin(qab);
      0 sin(qab) cos(qab)];
  
Qd40 = Qd43* Qd30;
Qd50=Qd54*Qd40;
Qd4g=Qd40*Qd0g;
Qd5g=Qd50*Qd0g;

%axis in local frames
ed1l=[1;0;0];
ed2l=[0;1;0];
ed3l=[0;
      0;
      1];
  
ed4l=[0;
      1;
      0];
ed5l=[0;
     1;
     0];
  
%link vector in local frame
ad3l=[0;
      0;
      -upper_leg_length];
   
ad4l=[0;
      0;
      -lower_leg_length];
         
%axis in global frames
eb1g=Qd30x*Qd0g*ed1l;
eb2g=Qd30x*Qd30y*Qd0g*ed2l;
eb3g =Qd30x*Qd30y*Qd30z*Qd0g*ed3l;
eb4g =Qd4g*ed4l;
eb5g =Qd5g*ed5l;

%link vector in global frame
ab1g=0;
ab2g=0;
ab3g = Qd3g*ad3l;
ab4g = Qd4g*ad4l;

%COM distances in base frame
cmb1g=0;
cmb2g=0;
cmb3g=ab3g/2;
cmb4g=ab4g/2;
cmb5g=Qd5g*foot_offset;

%I in global frame
I1=Qd30x*Qd0g*I1l*transpose(Qd30x*Qd0g);
I2=Qd30x*Qd30y*Qd0g*I2l*transpose(Qd30x*Qd30y*Qd0g);
I3=Qd30x*Qd30y*Qd30z*Qd0g*I3l*transpose(Qd30x*Qd30y*Qd30z*Qd0g);
I4=Qd4g*I4l*transpose(Qd4g);
I5=Qd5g*I5l*transpose(Qd5g);



end

== matlab function final_quadruped_080722_support_polygon/Model/Left Leg Front /Subsystem/MATLAB Function1 ==
  data: eb10g input; eb20g input; eb30g input; eb40g input; ab10g input; ab20g input; ab30g input; cmb4 input; cmb3 input; cmb5 input; eb50g input; ab40g input; hLF output; rhoLF output; cmb1 input; cmb2 input; I1 input; I2 input; I3 input; I4 input; I5 input; alpLF output; CMg input
function [hLF,rhoLF,alpLF] = fcn(eb10g,eb20g,eb30g, eb40g,ab10g,ab20g, ab30g, cmb4, cmb3, cmb5, eb50g, ab40g,cmb1,cmb2,I1,I2,I3,I4,I5, CMg)
%%
lower_leg_length = 10;
upper_leg_length = 10;
density = 1000;
foot_density=2000;
leg_radius = 0.75;
foot_x = 8;
foot_y = 6;
foot_z = 1;
m_ul=density*leg_radius*leg_radius*upper_leg_length*3.141592653589*0.01*0.01*0.01;
m_ll=density*leg_radius*leg_radius*lower_leg_length*3.141592653589*0.01*0.01*0.01;
m_foot=foot_density*foot_x*foot_y*foot_z*0.000001;
m1=0;
m2=0;
%%
scf=zeros(3,5);
sof=zeros(3,5);
rhoLF=zeros(3,5,5);
scf(:,1)=[0;0;0];
scf(:,2)=[0;0;0];
scf(:,3)=cmb3;
scf(:,4)=ab30g+cmb4;
scf(:,5)=ab30g+ab40g+cmb5;
sof(:,1)=[0;0;0];
sof(:,2)=[0;0;0];
sof(:,3)=[0;0;0];
sof(:,4)=ab30g;
sof(:,5)=ab30g+ab40g;
for i=1:5
    for j=1:5
        if j<i
rhoLF(:,j,i)=zeros(3,1);
        else
rhoLF(:,j,i)=scf(:,j)-sof(:,i);
        end
    end
end

c5=cmb5-CMg;
c4=cmb4-CMg;
c3=cmb3-CMg;
c2=cmb2-CMg;
c1=cmb1-CMg;

h1=m1*(cross(eb10g,rhoLF(:,1,1)))+m2*(cross(eb10g,rhoLF(:,2,1)))+m_ul*(cross(eb10g,rhoLF(:,3,1)))+m_ll*(cross(eb10g,rhoLF(:,4,1)))+m_foot*(cross(eb10g,rhoLF(:,5,1)));
h2=m2*(cross(eb20g,rhoLF(:,2,2)))+m_ul*(cross(eb20g,rhoLF(:,3,2)))+m_ll*(cross(eb20g,rhoLF(:,4,2)))+m_foot*(cross(eb20g,rhoLF(:,5,2)));
h3=(m_ul*cross(eb30g,rhoLF(:,3,3)))+(m_ll*cross(eb30g,rhoLF(:,4,3)))+(m_foot*cross(eb30g,rhoLF(:,5,3)));
h4=(m_ll*cross(eb40g,rhoLF(:,4,4)))+(m_foot*cross(eb40g,rhoLF(:,5,4)));
h5=m_foot*(cross(eb50g,rhoLF(:,5,5)));

hLF =[h1 h2 h3 h4 h5];

alp1=skewsymmetric(c1)*m1*cross(eb10g,rhoLF(:,1,1))+skewsymmetric(c2)*m2*cross(eb10g,rhoLF(:,2,1))+skewsymmetric(c3)*m_ul*cross(eb10g,rhoLF(:,3,1))+skewsymmetric(c4)*m_ll*cross(eb10g,rhoLF(:,4,1))+skewsymmetric(c5)*m_foot*cross(eb10g,rhoLF(:,5,1))+(I1+I2+I3+I4+I5)*eb10g;
alp2=skewsymmetric(c2)*m2*(cross(eb20g,rhoLF(:,2,2)))+skewsymmetric(c3)*m_ul*(cross(eb20g,rhoLF(:,3,2)))+skewsymmetric(c4)*m_ll*(cross(eb20g,rhoLF(:,4,2)))+skewsymmetric(c5)*m_foot*(cross(eb20g,rhoLF(:,5,2)))+(I2+I3+I4+I5)*eb20g;
alp3=skewsymmetric(c3)*m_ul*cross(eb30g,rhoLF(:,3,3))+skewsymmetric(c4)*m_ll*cross(eb30g,rhoLF(:,4,3))+skewsymmetric(c5)*m_foot*cross(eb30g,rhoLF(:,5,3))+(I3+I4+I5)*eb30g;
alp4=skewsymmetric(c4)*m_ll*cross(eb40g,rhoLF(:,4,4))+skewsymmetric(c5)*m_foot*cross(eb40g,rhoLF(:,5,4))+(I4+I5)*eb40g;
alp5=skewsymmetric(c5)*m_foot*cross(eb50g,rhoLF(:,5,5))+I5*eb50g;

alpLF=[alp1 alp2 alp3 alp4 alp5];



end
